simulink model "NewPlantPID (2)"  (R2025b)
settings: Solver=VariableStepAuto  StartTime=0.0  StopTime=1296  RelTol=1e-3
libraries: slpidlib x1
settings Model: Creator=suyas  LastModifiedBy=suyas

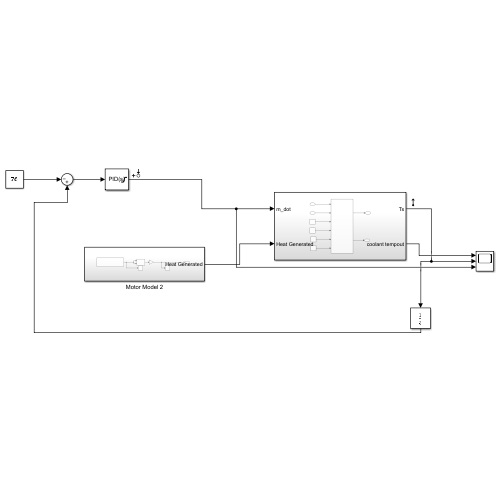
[thumbnail: Simulink's stored preview of the top-level diagram]
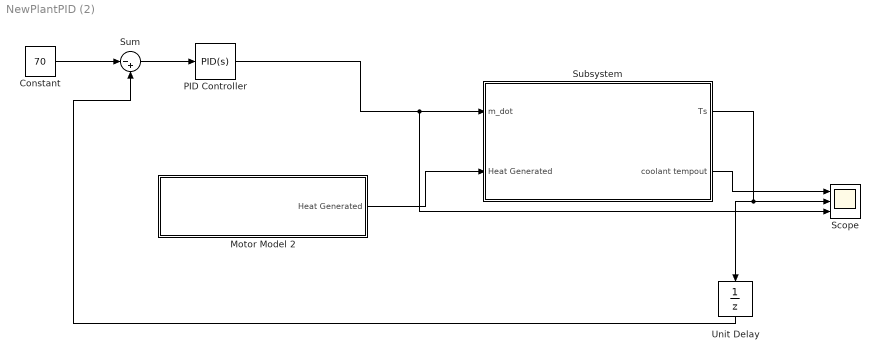
== system NewPlantPID (2) ==
  Constant : Constant  Value=70
  Motor Model 2 : Subsystem
  PID Controller : slpidlib/PID Controller  Controller=PID  Form=Ideal  TimeDomain=Continuous-time  UseExternalTs=off  SampleTime=-1  IntegratorMethod=Trapezoidal  FilterMethod=Trapezoidal  ControllerParametersSource=internal  P=-0.1  I=-0.5  UseKiTs=off  D=0  UseExternalDerivativeSource=off  N=20  UseFilter=on  TunerSelectOption=Transfer Function Based (PID Tuner App)  InitialConditionSource=internal  InitialConditionForIntegrator=0  InitialConditionForFilter=0  DifferentiatorICPrevScaledInput=0  ExternalReset=none  TrackingMode=off  Kt=1  LimitOutput=on  SatLimitsSource=internal  UpperSaturationLimit=0.267  LowerSaturationLimit=0  LinearizeAsGain=on  AntiWindupMode=back-calculation  Kb=100  LimitIntegrator=off  UpperIntegratorSaturationLimit=inf  LowerIntegratorSaturationLimit=-inf  POutMin=[]  POutMax=[]  IOutMin=[]  IOutMax=[]  DOutMin=[]  DOutMax=[]  NOutMin=[]  NOutMax=[]  SumOutMin=[]  SumOutMax=[]  SaturationOutMin=[]  SaturationOutMax=[]  PParamMin=[]  PParamMax=[]  IParamMin=[]  IParamMax=[]  DParamMin=[]  DParamMax=[]  NParamMin=[]  NParamMax=[]  KbParamMin=[]  KbParamMax=[]  KtParamMin=[]  KtParamMax=[]  KbOutMin=[]  KbOutMax=[]  KtOutMin=[]  KtOutMax=[]  IntegratorOutMin=[]  IntegratorOutMax=[]  FilterOutMin=[]  FilterOutMax=[]  SumI1OutMin=[]  SumI1OutMax=[]  SumI2OutMin=[]  SumI2OutMax=[]  SumI3OutMin=[]  SumI3OutMax=[]  SumI4OutMin=[]  SumI4OutMax=[]  SumDOutMin=[]  SumDOutMax=[]  DifferentiatorOutMin=[]  DifferentiatorOutMax=[]  FilterDiffOutCoefMin=[]  FilterDiffOutCoefMax=[]  ReciprocalOutMin=[]  ReciprocalOutMax=[]  SumDenOutMin=[]  SumDenOutMax=[]  SumNumOutMin=[]  SumNumOutMax=[]  DivideOutMin=[]  DivideOutMax=[]  UdiffTsProdOutMin=[]  UdiffTsProdOutMax=[]  NTsProdOutMin=[]  NTsProdOutMax=[]  UintegralTsProdOutMin=[]  UintegralTsProdOutMax=[]  UngainTsProdOutMin=[]  UngainTsProdOutMax=[]  ClampingZeroOutDataTypeStr=Inherit: Inherit via back propagation  ClampingZeroOutMin=[]  ClampingZeroOutMax=[]  FilterDenConstantOutDataTypeStr=Inherit: Inherit via back propagation  FilterDenConstantOutMin=[]  FilterDenConstantOutMax=[]  PCopyOutDataTypeStr=Inherit: Inherit via back propagation  PCopyOutMin=[]  PCopyOutMax=[]  NCopyOutDataTypeStr=Inherit: Inherit via back propagation  NCopyOutMin=[]  NCopyOutMax=[]  IntegratorContinuousStateAttributes=''  IntegratorStateMustResolveToSignalObject=off  IntegratorRTWStateStorageClass=Auto  FilterContinuousStateAttributes=''  FilterStateMustResolveToSignalObject=off  FilterRTWStateStorageClass=Auto  ParallelPVariant=Passthrough  IdealPVariant=InternalParameters  IVariant=InternalParameters  DVariant=InternalParameters  IntegratorVariant=Continuous  SatVariant=Enabled  AWVariant=BackCalculation  PCopyVariant=Disabled  TRVariant=Disabled  FdbkBlocksVariant=Forward  IdealPFdbkVariant=Disabled  SatFdbkVariant=Disabled  DerivativeFilterVariant=ContFilter  NVariant=InternalParameters  NCopyVariant=Disabled  FilterICVariant=InternalICsFilter  IntegratorICVariant=InternalICs  ExternalResetVariant=Disabled  TRSumVariant=Passthrough  SumFdbkVariant=Disabled  SumVariant=Sum_PID  TsampFilterVariant=InternalTs  TsampNgainVariant=Passthrough  TsampIntegralVariant=Disabled_SignalSpec  ExternalSaturationOutDataTypeStr=Inherit: Same as second input  DerivativeSourceVariant=ErrorSignal  PreIntVariant=InternalPreInt
  Scope : Scope  NumInputPorts=3
      settings: ActiveDisplayYMinimum=29.910881418499507  ActiveDisplayYMaximum=30.802067233504452
  Subsystem : Subsystem
  Sum : Sum  Inputs=|-+
  Unit Delay : UnitDelay  SampleTime=0.001  HasFrameUpgradeWarning=on
  wires:
  Motor Model 2/1(Heat Generated) -> Subsystem/2(Heat Generated)
  Subsystem/2(coolant tempout) -> Scope/1
  Constant/1 -> Sum/1
  Sum/1 -> PID Controller/1
  Subsystem/1(Ts) -> Scope/2, Unit Delay/1
  Unit Delay/1 -> Sum/2
  PID Controller/1 -> Scope/3, Subsystem/1(m_dot)

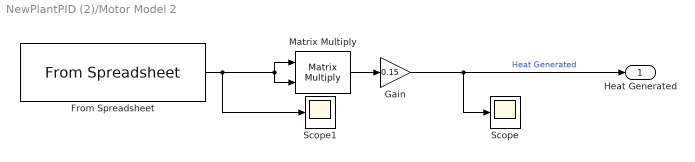
== system NewPlantPID (2)/Motor Model 2 ==
  From Spreadsheet : FromSpreadsheet  FileName=C:\Users\suyas\Downloads\expanded_data.xlsx  SampleTime=1
  Gain : Gain  Gain=0.15
  Matrix Multiply : Product  Multiplication=Matrix(*)
  Scope : Scope
      settings: ActiveDisplayYMinimum=-99.46168  ActiveDisplayYMaximum=895.15516  DataLoggingVariableName=ScopeData2
  Scope1 : Scope
      settings: ActiveDisplayYMinimum=-9.11588  ActiveDisplayYMaximum=81.93826
  Heat Generated : Outport
  wires:
  Matrix Multiply/1 -> Gain/1
  From Spreadsheet/1 -> Scope1/1, Matrix Multiply/2, Matrix Multiply/1
  Gain/1 -> Scope/1, Heat Generated/1  "Heat Generated"

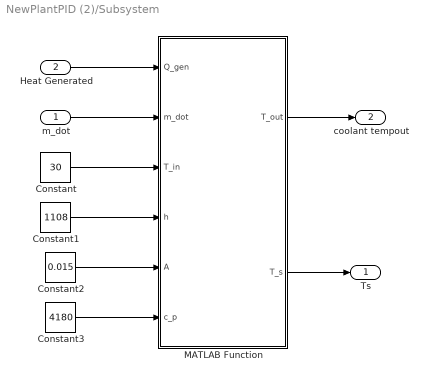
== system NewPlantPID (2)/Subsystem ==
  m_dot : Inport
  Heat Generated : Inport  Port=2
  Constant : Constant  Value=30
  Constant1 : Constant  Value=1108
  Constant2 : Constant  Value=0.015
  Constant3 : Constant  Value=4180
  MATLAB Function : MATLAB Function  TreatAsAtomicUnit=on
  Ts : Outport
  coolant tempout : Outport  Port=2
  wires:
  m_dot/1 -> MATLAB Function/2(m_dot)
  Heat Generated/1 -> MATLAB Function/1(Q_gen)
  Constant1/1 -> MATLAB Function/4(h)
  Constant2/1 -> MATLAB Function/5(A)
  Constant/1 -> MATLAB Function/3(T_in)
  Constant3/1 -> MATLAB Function/6(c_p)
  MATLAB Function/2(T_s) -> Ts/1
  MATLAB Function/1(T_out) -> coolant tempout/1

== matlab function NewPlantPID (2)/Subsystem/MATLAB Function ==
  data: Q_gen input; T_out output; m_dot input; T_in input; h input; A input; c_p input; T_s output
function [T_out, T_s] = CoolingJacket(Q_gen, m_dot, T_in, h, A, c_p)
%   Inputs...

% --- This is the fix ---
% Create a tiny, non-zero minimum flow rate to prevent divide-by-zero

% Use max() to "saturate" the m_dot at this minimum value.
% This is smooth and avoids the "if" discontinuity.
m_dot_safe = max(m_dot, 1e-6); 
% --- End of fix ---


% 1) Coolant outlet temperature (now numerically stable)
DeltaT = Q_gen / (m_dot_safe * c_p);
T_out = T_in + DeltaT;

% 2) Motor surface temperature
T_s = T_in + DeltaT/2 + Q_gen / (h * A);
end
